simulink model "PONG"  (R2018b)
settings: Solver=VariableStepAuto  StartTime=0.0  StopTime=10  RelTol=1e-3
libraries: simulink_extras x28
(part 1 of 3)
settings Model: SimulationMode=accelerator  NumberOfSteps=2  SnapshotBufferSize=100  SnapshotInterval=100  Creator=Baraghini Nicholas  LastModifiedBy=Baraghini Nicholas

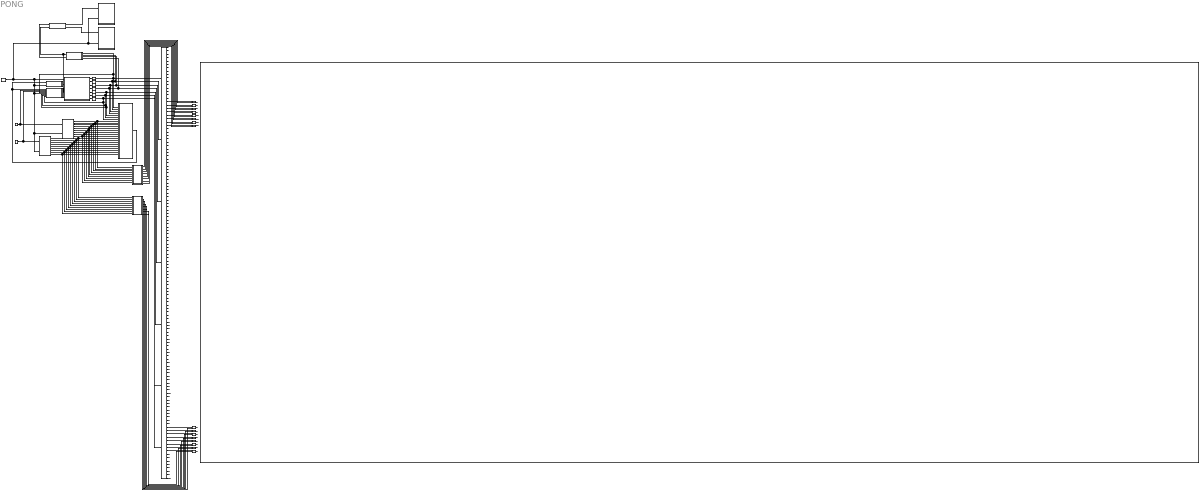
== system PONG ==
  Clock : simulink_extras/Flip Flops/Clock  period=1
  DECODER_7 bit : Subsystem  TreatAsAtomicUnit=on
  Horizontal Bounce : Subsystem  TreatAsAtomicUnit=on
  "LAMP_DISPLAY " : Subsystem  TreatAsAtomicUnit=on
  Logical Operator{,1..15} (16 alike) : Logic  Operator=OR  IconShape=distinctive  AllPortsSameDT=off  OutDataTypeStr=boolean
  Memory{,1..6} (7 alike) : Memory  InheritSampleTime=on
  "Next State " : Subsystem  TreatAsAtomicUnit=on
  Paddle Control : Subsystem  TreatAsAtomicUnit=on
  Paddle DEMUXER0 : Subsystem  TreatAsAtomicUnit=on
  Paddle DEMUXER1 : Subsystem  TreatAsAtomicUnit=on
  Paddle0 : Subsystem  TreatAsAtomicUnit=on
  Paddle1 : Subsystem  TreatAsAtomicUnit=on
  PointReset : Subsystem  TreatAsAtomicUnit=on
  Subsystem : Subsystem
  Subsystem2 : Subsystem
  Switch0 : Constant  OutDataTypeStr=boolean
  Switch1 : Constant  Value=0  OutDataTypeStr=boolean
  Vertical Bounce2 : Subsystem  TreatAsAtomicUnit=on
  Vertical Bounce3 : Subsystem  TreatAsAtomicUnit=on
  wires:
  "Next State "/1(A1) -> Memory6/1
  "Next State "/2(B1) -> Memory5/1
  "Next State "/3(C1) -> Memory4/1
  "Next State "/4(D1) -> Memory3/1
  "Next State "/5(E1) -> Memory2/1
  DECODER_7 bit/1(0000000) -> ?
  DECODER_7 bit/2("0000001 ") -> ?
  DECODER_7 bit/3(0000010) -> ?
  DECODER_7 bit/4(0000011) -> ?
  DECODER_7 bit/5(0000100) -> ?
  DECODER_7 bit/6(0000101) -> ?
  DECODER_7 bit/7(0000110) -> ?
  DECODER_7 bit/8(0000111) -> ?
  DECODER_7 bit/9(0001000) -> ?
  DECODER_7 bit/10(0001001) -> ?
  DECODER_7 bit/11(0001010) -> ?
  DECODER_7 bit/12(0001011) -> ?
  DECODER_7 bit/13(0001100) -> ?
  DECODER_7 bit/14(0001101) -> ?
  DECODER_7 bit/15(0001110) -> ?
  DECODER_7 bit/16(0001111) -> ?
  DECODER_7 bit/17(0010000) -> Logical Operator/1
  DECODER_7 bit/18(0010001) -> Logical Operator1/1
  DECODER_7 bit/19(0010010) -> Logical Operator2/1
  DECODER_7 bit/20(0010011) -> Logical Operator3/1
  DECODER_7 bit/21(0010100) -> Logical Operator4/1
  DECODER_7 bit/22(0010101) -> Logical Operator5/1
  DECODER_7 bit/23(0010110) -> Logical Operator6/1
  DECODER_7 bit/24(0010111) -> Logical Operator7/1
  DECODER_7 bit/25(0011000) -> ?
  DECODER_7 bit/26(0011001) -> ?
  DECODER_7 bit/27(0011010) -> ?
  DECODER_7 bit/28(0011011) -> ?
  DECODER_7 bit/29(0011100) -> ?
  DECODER_7 bit/30(0011101) -> ?
  DECODER_7 bit/31(0011110) -> ?
  DECODER_7 bit/32(0011111) -> ?
  DECODER_7 bit/33(0100000) -> ?
  DECODER_7 bit/34(0100001) -> ?
  DECODER_7 bit/35(0100010) -> ?
  DECODER_7 bit/36(0100011) -> ?
  DECODER_7 bit/37(0100100) -> ?
  DECODER_7 bit/38(0100110) -> ?
  DECODER_7 bit/39(0100111) -> ?
  DECODER_7 bit/40(0101000) -> ?
  DECODER_7 bit/41(0101001) -> ?
  DECODER_7 bit/42(0101010) -> ?
  DECODER_7 bit/43(0101011) -> ?
  DECODER_7 bit/44(0101100) -> ?
  DECODER_7 bit/45(0101101) -> ?
  DECODER_7 bit/46(0101110) -> ?
  DECODER_7 bit/47(0101111) -> ?
  DECODER_7 bit/48(0110000) -> ?
  DECODER_7 bit/49(0110001) -> ?
  DECODER_7 bit/50(0110010) -> ?
  DECODER_7 bit/51(0110011) -> ?
  DECODER_7 bit/52(0110100) -> ?
  DECODER_7 bit/53(0110101) -> ?
  DECODER_7 bit/54(0110110) -> ?
  DECODER_7 bit/55(0110111) -> ?
  DECODER_7 bit/56(0111000) -> ?
  DECODER_7 bit/57(0111001) -> ?
  DECODER_7 bit/58(0111010) -> ?
  DECODER_7 bit/59(0111011) -> ?
  DECODER_7 bit/60(0111100) -> ?
  DECODER_7 bit/61(0111101) -> ?
  DECODER_7 bit/62(0111110) -> ?
  DECODER_7 bit/63(0111111) -> ?
  DECODER_7 bit/64(0100101) -> ?
  DECODER_7 bit/65(1000000) -> ?
  DECODER_7 bit/66(1000001) -> ?
  DECODER_7 bit/67(1000010) -> ?
  DECODER_7 bit/68(1000011) -> ?
  DECODER_7 bit/69(1000100) -> ?
  DECODER_7 bit/70(1000101) -> ?
  DECODER_7 bit/71(1000110) -> ?
  DECODER_7 bit/72(1000111) -> ?
  DECODER_7 bit/73(1001000) -> ?
  DECODER_7 bit/74(1001001) -> ?
  DECODER_7 bit/75(1001010) -> ?
  DECODER_7 bit/76(1001011) -> ?
  DECODER_7 bit/77(1001100) -> ?
  DECODER_7 bit/78(1001101) -> ?
  DECODER_7 bit/79(1001110) -> ?
  DECODER_7 bit/80(1001111) -> ?
  DECODER_7 bit/81(1010000) -> ?
  DECODER_7 bit/82(1010001) -> ?
  DECODER_7 bit/83(1010010) -> ?
  DECODER_7 bit/84(1010011) -> ?
  DECODER_7 bit/85(1010100) -> ?
  DECODER_7 bit/86(1010101) -> ?
  DECODER_7 bit/87(1010110) -> ?
  DECODER_7 bit/88(1010111) -> ?
  DECODER_7 bit/89(1011000) -> ?
  DECODER_7 bit/90(1011001) -> ?
  DECODER_7 bit/91(1011010) -> ?
  DECODER_7 bit/92(1011011) -> ?
  DECODER_7 bit/113(1110000) -> Logical Operator8/1
  DECODER_7 bit/114(1110001) -> Logical Operator9/1
  DECODER_7 bit/115(1110010) -> Logical Operator10/1
  DECODER_7 bit/116(1110011) -> Logical Operator11/1
  DECODER_7 bit/117(1110100) -> Logical Operator12/1
  DECODER_7 bit/118(1110101) -> Logical Operator13/1
  DECODER_7 bit/119(1110110) -> Logical Operator14/1
  DECODER_7 bit/120(1110111) -> Logical Operator15/1
  Paddle0/1(PA) -> Paddle DEMUXER0/1(PA0), Paddle Control/8(PA)
  Paddle0/9(PC2) -> Paddle DEMUXER0/9(PC2), Paddle Control/16(PC2)
  Paddle0/8(PB2) -> Paddle DEMUXER0/8(PB2), Paddle Control/15(PB2)
  Paddle0/7(PA2) -> Paddle DEMUXER0/7(PA2), Paddle Control/14(PA2)
  Paddle0/2(PB) -> Paddle DEMUXER0/2(PB0), Paddle Control/9(PB)
  Paddle0/5(PB1) -> Paddle DEMUXER0/5(PB1), Paddle Control/12(PB1)
  Paddle1/1(PA) -> Paddle DEMUXER1/1(PA0), Paddle Control/17(1PA)
  Paddle1/3(PC) -> Paddle DEMUXER1/3(PC0), Paddle Control/19(1PC)
  Paddle1/4(PA1) -> Paddle DEMUXER1/4(PA1), Paddle Control/20(1PA1)
  Paddle1/5(PB1) -> Paddle DEMUXER1/5(PB1), Paddle Control/21(1PB1)
  Paddle1/9(PC2) -> Paddle DEMUXER1/9(PC2), Paddle Control/25(1PC2)
  Paddle Control/1(Check) -> Vertical Bounce3/1(Check), Horizontal Bounce/1(Check)
  "Next State "/6(F1) -> Memory1/1
  "Next State "/7(G1) -> Memory/1
  Paddle0/3(PC) -> Paddle DEMUXER0/3(PC0), Paddle Control/10(PC)
  Paddle0/4(PA1) -> Paddle DEMUXER0/4(PA1), Paddle Control/11(PA1)
  Paddle0/6(PC1) -> Paddle DEMUXER0/6(PC1), Paddle Control/13(PC1)
  Paddle1/2(PB) -> Paddle DEMUXER1/2(PB0), Paddle Control/18(1PB)
  Paddle1/6(PC1) -> Paddle DEMUXER1/6(PC1), Paddle Control/22(1PC1)
  Paddle1/7(PA2) -> Paddle DEMUXER1/7(PA2), Paddle Control/23(1PA2)
  Paddle1/8(PB2) -> Paddle DEMUXER1/8(PB2), Paddle Control/24(1PB2)
  Horizontal Bounce/1(HEnable) -> "Next State "/2(EN_Xball1)
  Switch0/1 -> Vertical Bounce3/2(Ctrl0), Paddle0/1(Controller)
  Switch1/1 -> Paddle1/1(Controller), Vertical Bounce3/3(Ctrl1)
  Logical Operator/1 -> ?
  Logical Operator8/1 -> ?
  Logical Operator9/1 -> ?
  Logical Operator10/1 -> ?
  Logical Operator11/1 -> ?
  Logical Operator12/1 -> ?
  Logical Operator13/1 -> ?
  Logical Operator14/1 -> ?
  Logical Operator15/1 -> ?
  Paddle DEMUXER0/1(000) -> Logical Operator/2
  Paddle DEMUXER0/2(001) -> Logical Operator1/2
  Paddle DEMUXER0/3(010) -> Logical Operator2/2
  Paddle DEMUXER0/4(011) -> Logical Operator3/2
  Paddle DEMUXER0/5(100) -> Logical Operator4/2
  Paddle DEMUXER0/6(101) -> Logical Operator5/2
  Paddle DEMUXER0/7(110) -> Logical Operator6/2
  Paddle DEMUXER0/8(111) -> Logical Operator7/2
  Paddle DEMUXER1/8(111) -> Logical Operator15/2
  Paddle DEMUXER1/7(110) -> Logical Operator14/2
  Paddle DEMUXER1/6(101) -> Logical Operator13/2
  Paddle DEMUXER1/1(000) -> Logical Operator8/2
  Paddle DEMUXER1/2(001) -> Logical Operator9/2
  Paddle DEMUXER1/3(010) -> Logical Operator10/2
  Paddle DEMUXER1/4(011) -> Logical Operator11/2
  Paddle DEMUXER1/5(100) -> Logical Operator12/2
  DECODER_7 bit/93("1011100 ") -> ?
  DECODER_7 bit/94(1011101) -> ?
  DECODER_7 bit/95(1011110) -> ?
  DECODER_7 bit/96(1011111) -> ?
  DECODER_7 bit/97(1100000) -> ?
  DECODER_7 bit/98(1100001) -> ?
  DECODER_7 bit/99(1100010) -> ?
  DECODER_7 bit/100(1100011) -> ?
  DECODER_7 bit/101(1100100) -> ?
  DECODER_7 bit/102(1100101) -> ?
  DECODER_7 bit/103(1100110) -> ?
  DECODER_7 bit/104(1100111) -> ?
  DECODER_7 bit/105(1101000) -> ?
  DECODER_7 bit/106(1101001) -> ?
  DECODER_7 bit/107(1101010) -> ?
  DECODER_7 bit/108(1101011) -> ?
  DECODER_7 bit/109(1101100) -> ?
  DECODER_7 bit/110(1101101) -> ?
  DECODER_7 bit/111(1101110) -> ?
  DECODER_7 bit/112(1101111) -> ?
  DECODER_7 bit/121(1111000) -> ?
  DECODER_7 bit/122(1111001) -> ?
  DECODER_7 bit/123(1111010) -> ?
  DECODER_7 bit/124(1111011) -> ?
  DECODER_7 bit/125(1111100) -> ?
  DECODER_7 bit/126(1111101) -> ?
  DECODER_7 bit/127(1111110) -> ?
  DECODER_7 bit/128(1111111) -> ?
  Logical Operator1/1 -> ?
  Logical Operator2/1 -> ?
  Logical Operator3/1 -> ?
  Logical Operator4/1 -> ?
  Logical Operator5/1 -> ?
  Logical Operator6/1 -> ?
  Logical Operator7/1 -> ?
  Vertical Bounce3/1(VEnable 1) -> "Next State "/3(EN_Yball1)
  Vertical Bounce3/2(VEnable 0) -> "Next State "/4(EN_Yball0)
  Memory/1 -> DECODER_7 bit/7(In7), Vertical Bounce3/8(G), Paddle Control/7(G)
  Memory1/1 -> DECODER_7 bit/6(In6), Vertical Bounce3/7(F), Paddle Control/6(F)
  Memory2/1 -> DECODER_7 bit/5(In5), Vertical Bounce3/6(E), Paddle Control/5(E)
  Memory3/1 -> PointReset/4(D), DECODER_7 bit/4(In4), Paddle Control/4(D)
  Memory4/1 -> PointReset/3(C), DECODER_7 bit/3(In3), Paddle Control/3(C)
  Memory5/1 -> DECODER_7 bit/2(In2), PointReset/2(B), Paddle Control/2(B)
  Memory6/1 -> Vertical Bounce3/4(A), PointReset/1(A), Paddle Control/1(A), DECODER_7 bit/1(In1)
  PointReset/1(PointReset) -> Vertical Bounce2/2(PointReset), "Next State "/5("EN_reset ")
  Vertical Bounce2/2(Point1) -> Subsystem2/1(EN)
  Vertical Bounce2/1(Point0) -> Subsystem/1(En)
  PointReset/2(Winner) -> Vertical Bounce2/1(Winner)
  Clock/1 -> Subsystem/2(CLK), Subsystem2/2(CLK), "Next State "/1(CLK 1), Paddle1/2(CLK), Paddle0/2(CLK), Vertical Bounce3/5(CLK), Horizontal Bounce/2(CLK)

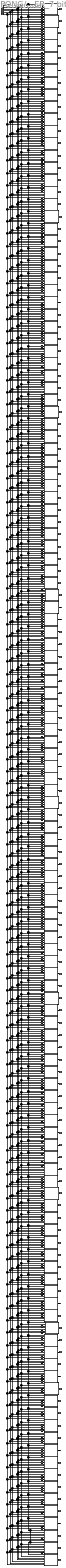
== system PONG/DECODER_7 bit ==
  In1 : Inport
  In2 : Inport  Port=2
  In3 : Inport  Port=3
  In4 : Inport  Port=4
  In5 : Inport  Port=5
  In6 : Inport  Port=6
  In7 : Inport  Port=7
  Logical Operator{,1..127} (128 alike) : Logic  Inputs=7  IconShape=distinctive  AllPortsSameDT=off  OutDataTypeStr=boolean
  NOT{,1..86,88..173,175..178,180..185,187..188,190..221,223..238,240..248,250..281,283..288,290,292..295,297..299,301,303..306,308..311,313..314,316,319..322,324..328,331..332,334..335,337..338,341..342,344,346,348..349,351,353..354,356..359,361..365,367..369,371..376,378..380,382..386,388,390..393,395,397..399,401..405,407..408,410,412..414,416..417,419..421,423..429,431,433..434,436..442,444..447,449..453,455..456,458..463,465..468,470..474,476..478,480..481,483..484,486..488,490..493,495,497..504,506..509,511..513} (448 alike) : Logic  Operator=NOT  IconShape=distinctive  AllPortsSameDT=off  OutDataTypeStr=boolean
  0000000 : Outport
  "0000001 " : Outport  Port=2
  0000010 : Outport  Port=3
  0000011 : Outport  Port=4
  0000100 : Outport  Port=5
  0000101 : Outport  Port=6
  0000110 : Outport  Port=7
  0000111 : Outport  Port=8
  0001000 : Outport  Port=9
  0001001 : Outport  Port=10
  0001010 : Outport  Port=11
  0001011 : Outport  Port=12
  0001100 : Outport  Port=13
  0001101 : Outport  Port=14
  0001110 : Outport  Port=15
  0001111 : Outport  Port=16
  0010000 : Outport  Port=17
  0010001 : Outport  Port=18
  0010010 : Outport  Port=19
  0010011 : Outport  Port=20
  0010100 : Outport  Port=21
  0010101 : Outport  Port=22
  0010110 : Outport  Port=23
  0010111 : Outport  Port=24
  0011000 : Outport  Port=25
  0011001 : Outport  Port=26
  0011010 : Outport  Port=27
  0011011 : Outport  Port=28
  0011100 : Outport  Port=29
  0011101 : Outport  Port=30
  0011110 : Outport  Port=31
  0011111 : Outport  Port=32
  0100000 : Outport  Port=33
  0100001 : Outport  Port=34
  0100010 : Outport  Port=35
  0100011 : Outport  Port=36
  0100100 : Outport  Port=37
  0100110 : Outport  Port=38
  0100111 : Outport  Port=39
  0101000 : Outport  Port=40
  0101001 : Outport  Port=41
  0101010 : Outport  Port=42
  0101011 : Outport  Port=43
  0101100 : Outport  Port=44
  0101101 : Outport  Port=45
  0101110 : Outport  Port=46
  0101111 : Outport  Port=47
  0110000 : Outport  Port=48
  0110001 : Outport  Port=49
  0110010 : Outport  Port=50
  0110011 : Outport  Port=51
  0110100 : Outport  Port=52
  0110101 : Outport  Port=53
  0110110 : Outport  Port=54
  0110111 : Outport  Port=55
  0111000 : Outport  Port=56
  0111001 : Outport  Port=57
  0111010 : Outport  Port=58
  0111011 : Outport  Port=59
  0111100 : Outport  Port=60
  0111101 : Outport  Port=61
  0111110 : Outport  Port=62
  0111111 : Outport  Port=63
  0100101 : Outport  Port=64
  1000000 : Outport  Port=65
  1000001 : Outport  Port=66
  1000010 : Outport  Port=67
  1000011 : Outport  Port=68
  1000100 : Outport  Port=69
  1000101 : Outport  Port=70
  1000110 : Outport  Port=71
  1000111 : Outport  Port=72
  1001000 : Outport  Port=73
  1001001 : Outport  Port=74
  1001010 : Outport  Port=75
  1001011 : Outport  Port=76
  1001100 : Outport  Port=77
  1001101 : Outport  Port=78
  1001110 : Outport  Port=79
  1001111 : Outport  Port=80
  1010000 : Outport  Port=81
  1010001 : Outport  Port=82
  1010010 : Outport  Port=83
  1010011 : Outport  Port=84
  1010100 : Outport  Port=85
  1010101 : Outport  Port=86
  1010110 : Outport  Port=87
  1010111 : Outport  Port=88
  1011000 : Outport  Port=89
  1011001 : Outport  Port=90
  1011010 : Outport  Port=91
  1011011 : Outport  Port=92
  "1011100 " : Outport  Port=93
  1011101 : Outport  Port=94
  1011110 : Outport  Port=95
  1011111 : Outport  Port=96
  1100000 : Outport  Port=97
  1100001 : Outport  Port=98
  1100010 : Outport  Port=99
  1100011 : Outport  Port=100
  1100100 : Outport  Port=101
  1100101 : Outport  Port=102
  1100110 : Outport  Port=103
  1100111 : Outport  Port=104
  1101000 : Outport  Port=105
  1101001 : Outport  Port=106
  1101010 : Outport  Port=107
  1101011 : Outport  Port=108
  1101100 : Outport  Port=109
  1101101 : Outport  Port=110
  1101110 : Outport  Port=111
  1101111 : Outport  Port=112
  1110000 : Outport  Port=113
  1110001 : Outport  Port=114
  1110010 : Outport  Port=115
  1110011 : Outport  Port=116
  1110100 : Outport  Port=117
  1110101 : Outport  Port=118
  1110110 : Outport  Port=119
  1110111 : Outport  Port=120
  1111000 : Outport  Port=121
  1111001 : Outport  Port=122
  1111010 : Outport  Port=123
  1111011 : Outport  Port=124
  1111100 : Outport  Port=125
  1111101 : Outport  Port=126
  1111110 : Outport  Port=127
  1111111 : Outport  Port=128
  wires:
  NOT/1 -> Logical Operator/1
  NOT1/1 -> Logical Operator/2
  NOT2/1 -> Logical Operator/3
  NOT3/1 -> Logical Operator/4
  NOT4/1 -> Logical Operator/5
  NOT5/1 -> Logical Operator/6
  NOT6/1 -> Logical Operator/7
  NOT7/1 -> Logical Operator1/1
  NOT8/1 -> Logical Operator1/2
  NOT9/1 -> Logical Operator1/3
  NOT10/1 -> Logical Operator1/4
  NOT11/1 -> Logical Operator1/5
  NOT12/1 -> Logical Operator1/6
  NOT17/1 -> Logical Operator2/5
  NOT13/1 -> Logical Operator2/1
  NOT14/1 -> Logical Operator2/2
  NOT15/1 -> Logical Operator2/3
  NOT16/1 -> Logical Operator2/4
  NOT19/1 -> Logical Operator2/7
  NOT23/1 -> Logical Operator3/5
  NOT18/1 -> Logical Operator3/1
  NOT20/1 -> Logical Operator3/2
  NOT21/1 -> Logical Operator3/3
  NOT22/1 -> Logical Operator3/4
  In7/1 -> Logical Operator1/7, NOT19/1, Logical Operator7/7, NOT50/1, NOT61/1, Logical Operator11/7, Logical Operator13/7, Logical Operator15/7, Logical Operator26/7, Logical Operator28/7, Logical Operator30/7, NOT132/1, NOT144/1, Logical Operator20/7, NOT163/1, Logical Operator54/7, Logical Operator59/7, Logical Operator35/7, Logical Operator37/7, Logical Operator39/7, NOT286/1, Logical Operator52/7, NOT165/1, NOT173/1, NOT183/1, Logical Operator44/7, NOT192/1, Logical Operator48/7, Logical Operator65/7, Logical Operator87/7, NOT451/1, Logical Operator67/7, NOT492/1, NOT500/1, Logical Operator74/7, Logical Operator83/7, NOT267/1, Logical Operator90/7, Logical Operator77/7, NOT316/1, Logical Operator79/7, NOT325/1, Logical Operator81/7, NOT402/1, NOT327/1, Logical Operator115/7, Logical Operator117/7, Logical Operator105/7, NOT356/1, Logical Operator107/7, NOT351/1, Logical Operator103/7, NOT342/1, NOT335/1, Logical Operator112/7, NOT288/1, Logical Operator110/7, NOT436/1, Logical Operator100/7, NOT426/1, Logical Operator97/7, NOT420/1, Logical Operator95/7, NOT413/1, Logical Operator93/7, NOT404/1, Logical Operator124/7, NOT393/1, Logical Operator122/7, NOT383/1, Logical Operator119/7, NOT373/1, Logical Operator114/7, NOT361/1, Logical Operator91/7, NOT306/1, NOT293/1, Logical Operator88/7, Logical Operator85/7, NOT200/1, NOT511/1, Logical Operator71/7, Logical Operator69/7, NOT483/1, NOT473/1, Logical Operator127/7, NOT461/1, Logical Operator125/7, Logical Operator109/7, NOT439/1, NOT348/1, NOT471/1, NOT199/1, Logical Operator46/7, Logical Operator57/7, Logical Operator55/7, NOT127/1, Logical Operator50/7, Logical Operator41/7, NOT276/1, NOT269/1, NOT260/1, NOT250/1, Logical Operator63/7, NOT238/1, Logical Operator61/7, NOT228/1, NOT216/1, NOT203/1, Logical Operator33/7, NOT248/1, Logical Operator24/7, Logical Operator22/7, NOT154/1, Logical Operator32/7, NOT122/1, NOT110/1, NOT97/1, Logical Operator18/7, NOT86/1, NOT79/1, NOT70/1, Logical Operator9/7, NOT41/1, Logical Operator5/7, NOT30/1, Logical Operator3/7, NOT6/1
  NOT25/1 -> Logical Operator4/2
  NOT26/1 -> Logical Operator4/3
  NOT27/1 -> Logical Operator4/4
  NOT24/1 -> Logical Operator4/1
  NOT29/1 -> Logical Operator4/6
  NOT30/1 -> Logical Operator4/7
  NOT31/1 -> Logical Operator5/2
  NOT32/1 -> Logical Operator5/3
  NOT33/1 -> Logical Operator5/4
  NOT28/1 -> Logical Operator5/1
  NOT35/1 -> Logical Operator5/6
  NOT36/1 -> Logical Operator6/2
  NOT37/1 -> Logical Operator6/3
  NOT38/1 -> Logical Operator6/4
  NOT34/1 -> Logical Operator6/1
  NOT41/1 -> Logical Operator6/7
  NOT40/1 -> Logical Operator7/2
  NOT42/1 -> Logical Operator7/3
  NOT43/1 -> Logical Operator7/4
  NOT39/1 -> Logical Operator7/1
  NOT45/1 -> Logical Operator8/2
  NOT46/1 -> Logical Operator8/3
  NOT48/1 -> Logical Operator8/5
  NOT44/1 -> Logical Operator8/1
  NOT49/1 -> Logical Operator8/6
  NOT50/1 -> Logical Operator8/7
  NOT51/1 -> Logical Operator9/2
  NOT52/1 -> Logical Operator9/3
  NOT54/1 -> Logical Operator9/5
  NOT47/1 -> Logical Operator9/1
  NOT55/1 -> Logical Operator9/6
  NOT56/1 -> Logical Operator10/2
  NOT57/1 -> Logical Operator10/3
  NOT59/1 -> Logical Operator10/5
  NOT53/1 -> Logical Operator10/1
  NOT61/1 -> Logical Operator10/7
  NOT60/1 -> Logical Operator11/2
  NOT62/1 -> Logical Operator11/3
  NOT64/1 -> Logical Operator11/5
  NOT58/1 -> Logical Operator11/1
  NOT65/1 -> Logical Operator12/2
  NOT66/1 -> Logical Operator12/3
  NOT63/1 -> Logical Operator12/1
  NOT69/1 -> Logical Operator12/6
  NOT70/1 -> Logical Operator12/7
  NOT68/1 -> Logical Operator13/2
  NOT71/1 -> Logical Operator13/3
  NOT67/1 -> Logical Operator13/1
  NOT74/1 -> Logical Operator13/6
  NOT73/1 -> Logical Operator14/2
  NOT75/1 -> Logical Operator14/3
  NOT72/1 -> Logical Operator14/1
  NOT79/1 -> Logical Operator14/7
  NOT77/1 -> Logical Operator15/2
  NOT78/1 -> Logical Operator15/3
  NOT76/1 -> Logical Operator15/1
  NOT81/1 -> Logical Operator16/2
  NOT83/1 -> Logical Operator16/4
  NOT84/1 -> Logical Operator16/5
  NOT80/1 -> Logical Operator16/1
  NOT85/1 -> Logical Operator16/6
  NOT86/1 -> Logical Operator16/7
  NOT97/1 -> Logical Operator25/7
  NOT89/1 -> Logical Operator18/5
  NOT160/1 -> Logical Operator24/1
  NOT144/1 -> Logical Operator19/7
  NOT135/1 -> Logical Operator19/1
  NOT141/1 -> Logical Operator19/5
  NOT138/1 -> Logical Operator19/2
  NOT150/1 -> Logical Operator22/1
  NOT161/1 -> Logical Operator24/2
  NOT151/1 -> Logical Operator22/2
  NOT163/1 -> Logical Operator23/7
  NOT156/1 -> Logical Operator23/1
  NOT158/1 -> Logical Operator22/6
  NOT137/1 -> Logical Operator32/6
  NOT128/1 -> Logical Operator32/1
  NOT136/1 -> Logical Operator32/5
  NOT133/1 -> Logical Operator32/2
  NOT132/1 -> Logical Operator31/7
  NOT125/1 -> Logical Operator31/1
  NOT129/1 -> Logical Operator31/5
  NOT115/1 -> Logical Operator28/6
  NOT107/1 -> Logical Operator28/1
  NOT147/1 -> Logical Operator20/5
  NOT143/1 -> Logical Operator20/2
  NOT146/1 -> Logical Operator21/1
  NOT122/1 -> Logical Operator29/7
  NOT88/1 -> Logical Operator18/4
  NOT113/1 -> Logical Operator28/4
  NOT126/1 -> Logical Operator31/2
  NOT104/1 -> Logical Operator27/2
  NOT110/1 -> Logical Operator27/7
  NOT108/1 -> Logical Operator27/6
  NOT140/1 -> Logical Operator20/1
  NOT103/1 -> Logical Operator27/1
  NOT99/1 -> Logical Operator26/2
  NOT111/1 -> Logical Operator28/2
  NOT101/1 -> Logical Operator26/4
  NOT96/1 -> Logical Operator26/1
  NOT114/1 -> Logical Operator29/1
  NOT157/1 -> Logical Operator23/2
  NOT118/1 -> Logical Operator29/4
  NOT102/1 -> Logical Operator26/5
  NOT116/1 -> Logical Operator29/2
  NOT90/1 -> Logical Operator18/6
  NOT164/1 -> Logical Operator18/2
  NOT94/1 -> Logical Operator25/4
  NOT91/1 -> Logical Operator25/1
  NOT92/1 -> Logical Operator25/2
  NOT95/1 -> Logical Operator25/5
  NOT152/1 -> Logical Operator21/6
  NOT148/1 -> Logical Operator21/2
  NOT130/1 -> Logical Operator31/6
  NOT121/1 -> Logical Operator30/2
  NOT154/1 -> Logical Operator21/7
  NOT124/1 -> Logical Operator30/4
  NOT153/1 -> Logical Operator18/1
  NOT119/1 -> Logical Operator30/1
  NOT106/1 -> Logical Operator27/4
  NOT203/1 -> Logical Operator43/7
  NOT226/1 -> Logical Operator17/5
  NOT276/1 -> Logical Operator40/7
  NOT273/1 -> Logical Operator40/4
  NOT266/1 -> Logical Operator39/1
  NOT274/1 -> Logical Operator40/5
  NOT117/1 -> Logical Operator52/1
  NOT185/1 -> Logical Operator44/5
  NOT142/1 -> Logical Operator52/6
  NOT176/1 -> Logical Operator57/5
  NOT177/1 -> Logical Operator57/6
  NOT169/1 -> Logical Operator57/1
  NOT188/1 -> Logical Operator46/1
  NOT175/1 -> Logical Operator42/1
  NOT183/1 -> Logical Operator42/7
  NOT181/1 -> Logical Operator42/5
  NOT237/1 -> Logical Operator17/6
  NOT197/1 -> Logical Operator48/1
  NOT278/1 -> Logical Operator41/5
  NOT286/1 -> Logical Operator49/7
  NOT155/1 -> Logical Operator55/1
  NOT166/1 -> Logical Operator55/4
  NOT123/1 -> Logical Operator33/5
  NOT192/1 -> Logical Operator45/7
  NOT190/1 -> Logical Operator45/6
  NOT284/1 -> Logical Operator49/5
  NOT281/1 -> Logical Operator49/1
  NOT280/1 -> Logical Operator41/6
  NOT100/1 -> Logical Operator50/5
  NOT283/1 -> Logical Operator49/4
  NOT172/1 -> Logical Operator56/6
  NOT139/1 -> Logical Operator53/1
  NOT285/1 -> Logical Operator50/1
  NOT184/1 -> Logical Operator45/1
  NOT105/1 -> Logical Operator51/1
  NOT165/1 -> Logical Operator53/7
  NOT127/1 -> Logical Operator51/7
  NOT277/1 -> Logical Operator41/4
  NOT120/1 -> Logical Operator51/6
  NOT134/1 -> Logical Operator52/4
  NOT245/1 -> Logical Operator34/3
  NOT250/1 -> Logical Operator34/7
  NOT241/1 -> Logical Operator34/1
  NOT247/1 -> Logical Operator34/5
  NOT193/1 -> Logical Operator47/1
  NOT256/1 -> Logical Operator37/1
  NOT261/1 -> Logical Operator37/3
  NOT265/1 -> Logical Operator38/3
  NOT269/1 -> Logical Operator38/7
  NOT262/1 -> Logical Operator38/1
  NOT264/1 -> Logical Operator37/6
  NOT243/1 -> Logical Operator63/6
  NOT234/1 -> Logical Operator63/1
  NOT149/1 -> Logical Operator53/4
  NOT242/1 -> Logical Operator63/5
  NOT199/1 -> Logical Operator47/7
  NOT238/1 -> Logical Operator62/7
  NOT231/1 -> Logical Operator62/1
  NOT235/1 -> Logical Operator62/5
  NOT233/1 -> Logical Operator62/3
  NOT98/1 -> Logical Operator50/4
  NOT240/1 -> Logical Operator63/3
  NOT221/1 -> Logical Operator59/6
  NOT213/1 -> Logical Operator59/1
  NOT253/1 -> Logical Operator35/5
  NOT252/1 -> Logical Operator36/1
  NOT228/1 -> Logical Operator60/7
  NOT93/1 -> Logical Operator33/4
  NOT219/1 -> Logical Operator59/4
  NOT191/1 -> Logical Operator41/1
  NOT216/1 -> Logical Operator58/7
  NOT214/1 -> Logical Operator58/6
  NOT246/1 -> Logical Operator35/1
  NOT209/1 -> Logical Operator58/1
  NOT180/1 -> Logical Operator44/1
  NOT279/1 -> Logical Operator33/3
  NOT211/1 -> Logical Operator58/3
  NOT206/1 -> Logical Operator54/3
  NOT112/1 -> Logical Operator51/4
  NOT207/1 -> Logical Operator54/4
  NOT202/1 -> Logical Operator54/1
  NOT82/1 -> Logical Operator17/1
  NOT220/1 -> Logical Operator60/1
  NOT224/1 -> Logical Operator60/4
  NOT223/1 -> Logical Operator60/3
  NOT208/1 -> Logical Operator54/5
  NOT159/1 -> Logical Operator33/6
  NOT173/1 -> Logical Operator56/7
  NOT196/1 -> Logical Operator43/4
  NOT195/1 -> Logical Operator46/6
  NOT251/1 -> Logical Operator35/3
  NOT271/1 -> Logical Operator40/1
  NOT171/1 -> Logical Operator43/1
  NOT268/1 -> Logical Operator39/3
  NOT218/1 -> Logical Operator59/3
  NOT201/1 -> Logical Operator43/5
  NOT248/1 -> Logical Operator17/7
  NOT255/1 -> Logical Operator36/3
  NOT258/1 -> Logical Operator36/6
  NOT236/1 -> Logical Operator62/6
  NOT229/1 -> Logical Operator61/3
  NOT275/1 -> Logical Operator40/6
  NOT260/1 -> Logical Operator36/7
  NOT230/1 -> Logical Operator61/4
  NOT259/1 -> Logical Operator33/1
  NOT170/1 -> Logical Operator56/5
  NOT204/1 -> Logical Operator17/3
  NOT187/1 -> Logical Operator43/3
  NOT215/1 -> Logical Operator17/4
  NOT225/1 -> Logical Operator61/1
  NOT212/1 -> Logical Operator58/4
  NOT167/1 -> Logical Operator56/1
  NOT449/1 -> Logical Operator64/5
  NOT498/1 -> Logical Operator72/5
  NOT337/1 -> Logical Operator117/5
  In1/1 -> NOT/1, NOT7/1, Logical Operator70/1, Logical Operator71/1, Logical Operator72/1, Logical Operator74/1, Logical Operator82/1, Logical Operator83/1, Logical Operator84/1, Logical Operator85/1, Logical Operator86/1, Logical Operator88/1, Logical Operator89/1, Logical Operator77/1, Logical Operator78/1, Logical Operator79/1, Logical Operator80/1, Logical Operator81/1, Logical Operator73/1, Logical Operator91/1, Logical Operator102/1, Logical Operator114/1, Logical Operator118/1, Logical Operator119/1, Logical Operator122/1, Logical Operator123/1, Logical Operator124/1, Logical Operator92/1, Logical Operator93/1, Logical Operator94/1, Logical Operator95/1, Logical Operator96/1, Logical Operator97/1, Logical Operator99/1, Logical Operator100/1, Logical Operator108/1, Logical Operator110/1, Logical Operator111/1, Logical Operator112/1, Logical Operator113/1, Logical Operator117/1, Logical Operator101/1, Logical Operator103/1, Logical Operator104/1, Logical Operator107/1, Logical Operator106/1, Logical Operator105/1, Logical Operator116/1, Logical Operator115/1, Logical Operator121/1, Logical Operator75/1, Logical Operator90/1, Logical Operator69/1, Logical Operator68/1, Logical Operator67/1, Logical Operator66/1, Logical Operator127/1, Logical Operator126/1, Logical Operator125/1, Logical Operator120/1, Logical Operator109/1, Logical Operator98/1, Logical Operator87/1, Logical Operator76/1, Logical Operator65/1, Logical Operator64/1, NOT197/1, NOT193/1, NOT188/1, NOT184/1, NOT180/1, NOT175/1, NOT169/1, NOT167/1, NOT155/1, NOT139/1, NOT117/1, NOT105/1, NOT285/1, NOT281/1, NOT191/1, NOT271/1, NOT266/1, NOT262/1, NOT256/1, NOT252/1, NOT246/1, NOT241/1, NOT234/1, NOT231/1, NOT225/1, NOT220/1, NOT213/1, NOT209/1, NOT202/1, NOT171/1, NOT259/1, NOT82/1, NOT160/1, NOT156/1, NOT150/1, NOT146/1, NOT140/1, NOT135/1, NOT128/1, NOT125/1, NOT119/1, NOT114/1, NOT107/1, NOT103/1, NOT96/1, NOT91/1, NOT153/1, NOT80/1, NOT76/1, NOT72/1, NOT67/1, NOT63/1, NOT58/1, NOT53/1, NOT47/1, NOT44/1, NOT39/1, NOT34/1, NOT28/1, NOT24/1, NOT18/1, NOT13/1
  NOT497/1 -> Logical Operator72/4
  NOT401/1 -> Logical Operator92/5
  NOT404/1 -> Logical Operator92/7
  NOT427/1 -> Logical Operator100/4
  NOT288/1 -> Logical Operator111/7
  NOT327/1 -> Logical Operator113/7
  NOT433/1 -> Logical Operator108/4
  NOT145/1 -> Logical Operator110/5
  NOT431/1 -> Logical Operator100/6
  NOT434/1 -> Logical Operator108/5
  NOT351/1 -> Logical Operator104/7
  In2/1 -> NOT8/1, NOT14/1, NOT20/1, NOT25/1, NOT36/1, NOT40/1, NOT45/1, NOT51/1, NOT60/1, NOT65/1, NOT68/1, NOT73/1, NOT77/1, NOT81/1, NOT164/1, NOT92/1, NOT99/1, NOT116/1, NOT126/1, NOT133/1, NOT143/1, NOT148/1, NOT151/1, NOT157/1, NOT161/1, Logical Operator17/2, Logical Operator33/2, Logical Operator43/2, Logical Operator54/2, Logical Operator58/2, Logical Operator59/2, Logical Operator61/2, Logical Operator36/2, Logical Operator38/2, Logical Operator40/2, Logical Operator49/2, Logical Operator52/2, Logical Operator53/2, Logical Operator55/2, Logical Operator56/2, Logical Operator57/2, Logical Operator44/2, Logical Operator45/2, Logical Operator46/2, Logical Operator47/2, Logical Operator48/2, NOT109/1, NOT493/1, NOT301/1, NOT358/1, NOT403/1, NOT440/1, NOT445/1, NOT450/1, NOT455/1, NOT462/1, NOT467/1, NOT472/1, NOT477/1, NOT480/1, NOT486/1, NOT490/1, NOT495/1, NOT326/1, NOT506/1, NOT513/1, NOT178/1, NOT232/1, NOT263/1, NOT287/1, NOT305/1, NOT309/1, NOT313/1, NOT319/1, NOT324/1, Logical Operator73/2, Logical Operator91/2, Logical Operator102/2, Logical Operator114/2, Logical Operator122/2, Logical Operator123/2, Logical Operator92/2, Logical Operator93/2, Logical Operator94/2, Logical Operator95/2, Logical Operator96/2, Logical Operator97/2, Logical Operator99/2, Logical Operator100/2, Logical Operator108/2, Logical Operator110/2, Logical Operator111/2, Logical Operator112/2, Logical Operator113/2, Logical Operator115/2, Logical Operator116/2, Logical Operator117/2, Logical Operator101/2, Logical Operator103/2, Logical Operator104/2, Logical Operator105/2, Logical Operator107/2, Logical Operator106/2, Logical Operator124/2, Logical Operator121/2, Logical Operator119/2, Logical Operator118/2, NOT299/1, NOT294/1, NOT205/1, Logical Operator42/2, Logical Operator51/2, Logical Operator50/2, Logical Operator41/2, Logical Operator39/2, Logical Operator37/2, Logical Operator35/2, Logical Operator34/2, Logical Operator63/2, Logical Operator62/2, Logical Operator60/2, NOT138/1, NOT121/1, NOT111/1, NOT104/1, NOT56/1, NOT31/1, NOT1/1
  NOT341/1 -> Logical Operator101/5
  NOT334/1 -> Logical Operator116/6
  NOT392/1 -> Logical Operator73/6
  NOT305/1 -> Logical Operator77/2
  NOT297/1 -> Logical Operator90/5
  NOT298/1 -> Logical Operator90/6
  NOT324/1 -> Logical Operator81/2
  NOT306/1 -> Logical Operator75/7
  NOT299/1 -> Logical Operator75/2
  NOT303/1 -> Logical Operator75/5
  NOT460/1 -> Logical Operator64/6
  NOT272/1 -> Logical Operator88/4
  NOT198/1 -> Logical Operator65/5
  NOT316/1 -> Logical Operator78/7
  NOT263/1 -> Logical Operator88/2
  NOT495/1 -> Logical Operator72/2
  NOT309/1 -> Logical Operator78/2
  NOT314/1 -> Logical Operator78/6
  NOT509/1 -> Logical Operator82/5
  NOT504/1 -> Logical Operator74/6
  NOT168/1 -> Logical Operator83/5
  NOT508/1 -> Logical Operator82/4
  NOT292/1 -> Logical Operator89/6
  NOT319/1 -> Logical Operator80/2
  NOT232/1 -> Logical Operator86/2
  NOT295/1 -> Logical Operator112/4
  NOT513/1 -> Logical Operator83/2
  NOT205/1 -> Logical Operator85/2
  NOT270/1 -> Logical Operator91/5
  NOT267/1 -> Logical Operator86/7
  NOT200/1 -> Logical Operator84/7
  NOT501/1 -> Logical Operator74/4
  NOT217/1 -> Logical Operator85/4
  NOT287/1 -> Logical Operator89/2
  NOT468/1 -> Logical Operator66/3
  NOT473/1 -> Logical Operator66/7
  NOT470/1 -> Logical Operator66/5
  NOT467/1 -> Logical Operator66/2
  NOT484/1 -> Logical Operator69/3
  NOT490/1 -> Logical Operator71/2
  NOT480/1 -> Logical Operator69/2
  NOT436/1 -> Logical Operator108/7
  NOT492/1 -> Logical Operator70/7
  NOT487/1 -> Logical Operator69/6
  In5/1 -> NOT17/1, NOT23/1, Logical Operator4/5, Logical Operator6/5, Logical Operator7/5, NOT48/1, NOT54/1, NOT59/1, NOT64/1, Logical Operator12/5, Logical Operator15/5, NOT89/1, NOT102/1, Logical Operator27/5, Logical Operator29/5, Logical Operator21/5, Logical Operator24/5, NOT226/1, NOT201/1, NOT208/1, Logical Operator60/5, Logical Operator61/5, NOT235/1, NOT253/1, Logical Operator36/5, Logical Operator37/5, Logical Operator38/5, Logical Operator39/5, NOT274/1, NOT278/1, NOT100/1, Logical Operator51/5, Logical Operator52/5, Logical Operator53/5, NOT170/1, NOT176/1, NOT181/1, NOT185/1, Logical Operator45/5, Logical Operator46/5, Logical Operator47/5, NOT449/1, NOT198/1, NOT331/1, Logical Operator98/5, Logical Operator120/5, Logical Operator125/5, NOT458/1, NOT465/1, NOT470/1, NOT476/1, Logical Operator68/5, Logical Operator69/5, Logical Operator71/5, NOT509/1, NOT168/1, Logical Operator85/5, Logical Operator88/5, NOT297/1, NOT303/1, NOT308/1, Logical Operator78/5, Logical Operator81/5, NOT382/1, NOT270/1, NOT359/1, NOT365/1, Logical Operator119/5, Logical Operator121/5, Logical Operator122/5, NOT390/1, NOT397/1, NOT401/1, Logical Operator95/5, Logical Operator96/5, Logical Operator97/5, NOT424/1, NOT428/1, NOT434/1, Logical Operator111/5, Logical Operator113/5, Logical Operator115/5, NOT341/1, NOT344/1, Logical Operator104/5, Logical Operator105/5, Logical Operator107/5, Logical Operator106/5, NOT337/1, NOT332/1, Logical Operator112/5, NOT145/1, Logical Operator94/5, NOT407/1, Logical Operator118/5, Logical Operator80/5, Logical Operator79/5, NOT290/1, Logical Operator86/5, Logical Operator84/5, NOT502/1, NOT498/1, Logical Operator70/5, Logical Operator109/5, NOT385/1, Logical Operator48/5, Logical Operator55/5, NOT284/1, NOT247/1, NOT242/1, Logical Operator59/5, Logical Operator58/5, NOT123/1, Logical Operator23/5, Logical Operator22/5, NOT147/1, NOT141/1, NOT136/1, NOT129/1, Logical Operator30/5, Logical Operator28/5, NOT95/1, NOT84/1, Logical Operator14/5, Logical Operator13/5, Logical Operator5/5, NOT11/1, NOT4/1
  NOT294/1 -> Logical Operator90/2
  NOT413/1 -> Logical Operator94/7
  NOT428/1 -> Logical Operator100/5
  NOT425/1 -> Logical Operator99/6
  NOT391/1 -> Logical Operator123/6
  NOT408/1 -> Logical Operator94/3
  NOT402/1 -> Logical Operator73/7
  NOT359/1 -> Logical Operator102/5
  NOT374/1 -> Logical Operator119/3
  NOT328/1 -> Logical Operator115/4
  NOT419/1 -> Logical Operator97/3
  NOT349/1 -> Logical Operator104/6
  NOT354/1 -> Logical Operator102/4
  NOT353/1 -> Logical Operator105/6
  NOT502/1 -> Logical Operator74/5
  NOT321/1 -> Logical Operator91/6
  NOT335/1 -> Logical Operator116/7
  NOT379/1 -> Logical Operator121/3
  NOT380/1 -> Logical Operator121/4
  NOT365/1 -> Logical Operator114/5
  NOT210/1 -> Logical Operator111/4
  NOT363/1 -> Logical Operator114/3
  NOT371/1 -> Logical Operator118/6
  NOT507/1 -> Logical Operator91/4
  NOT375/1 -> Logical Operator119/4
  NOT383/1 -> Logical Operator121/7
  NOT342/1 -> Logical Operator101/7
  NOT348/1 -> Logical Operator76/7
  NOT395/1 -> Logical Operator124/3
  NOT378/1 -> Logical Operator119/6
  NOT407/1 -> Logical Operator93/5
  NOT512/1 -> Logical Operator110/4
  NOT326/1 -> Logical Operator74/2
  NOT390/1 -> Logical Operator123/5
  NOT393/1 -> Logical Operator123/7
  NOT308/1 -> Logical Operator77/5
  NOT398/1 -> Logical Operator124/6
  NOT356/1 -> Logical Operator106/7
  NOT488/1 -> Logical Operator70/3
  NOT397/1 -> Logical Operator124/5
  NOT310/1 -> Logical Operator113/4
  NOT420/1 -> Logical Operator96/7
  NOT417/1 -> Logical Operator96/3
  NOT429/1 -> Logical Operator91/3
  NOT257/1 -> Logical Operator111/6
  NOT368/1 -> Logical Operator118/3
  NOT466/1 -> Logical Operator127/6
  NOT244/1 -> Logical Operator86/4
  NOT465/1 -> Logical Operator127/5
  NOT325/1 -> Logical Operator80/7
  NOT462/1 -> Logical Operator127/2
  NOT461/1 -> Logical Operator126/7
  NOT458/1 -> Logical Operator126/5
  NOT455/1 -> Logical Operator126/2
  NOT386/1 -> Logical Operator122/4
  NOT456/1 -> Logical Operator126/3
  NOT162/1 -> Logical Operator83/4
  NOT442/1 -> Logical Operator109/4
  NOT463/1 -> Logical Operator127/3
  NOT444/1 -> Logical Operator109/6
  NOT440/1 -> Logical Operator109/2
  NOT182/1 -> Logical Operator84/4
  NOT474/1 -> Logical Operator67/3
  NOT476/1 -> Logical Operator67/5
  NOT338/1 -> Logical Operator117/6
  NOT472/1 -> Logical Operator67/2
  NOT399/1 -> Logical Operator92/3
  NOT414/1 -> Logical Operator95/3
  NOT451/1 -> Logical Operator120/7
  NOT503/1 -> Logical Operator65/3
  NOT131/1 -> Logical Operator65/4
  NOT477/1 -> Logical Operator68/2
  NOT459/1 -> Logical Operator126/6
  NOT478/1 -> Logical Operator68/3
  NOT439/1 -> Logical Operator98/7
  NOT437/1 -> Logical Operator98/6
  NOT388/1 -> Logical Operator123/3
  NOT358/1 -> Logical Operator87/2
  NOT412/1 -> Logical Operator98/3
  NOT367/1 -> Logical Operator87/3
  NOT382/1 -> Logical Operator73/5
  NOT361/1 -> Logical Operator102/7
  NOT194/1 -> Logical Operator84/6
  NOT511/1 -> Logical Operator82/7
  NOT178/1 -> Logical Operator84/2
  NOT424/1 -> Logical Operator99/5
  NOT423/1 -> Logical Operator99/4
  NOT426/1 -> Logical Operator99/7
  NOT410/1 -> Logical Operator94/6
  NOT486/1 -> Logical Operator70/2
  NOT344/1 -> Logical Operator103/5
  NOT446/1 -> Logical Operator120/3
  NOT385/1 -> Logical Operator87/5
  NOT445/1 -> Logical Operator120/2
  NOT493/1 -> Logical Operator65/2
  NOT322/1 -> Logical Operator76/4
  NOT320/1 -> Logical Operator79/6
  NOT491/1 -> Logical Operator71/3
  NOT331/1 -> Logical Operator76/5
  NOT447/1 -> Logical Operator120/4
  NOT373/1 -> Logical Operator118/7
  NOT369/1 -> Logical Operator118/4
  NOT376/1 -> Logical Operator87/4
  NOT254/1 -> Logical Operator65/6
  NOT293/1 -> Logical Operator89/7
  NOT372/1 -> Logical Operator73/4
  NOT109/1 -> Logical Operator64/2
  NOT346/1 -> Logical Operator102/3
  NOT405/1 -> Logical Operator93/3
  NOT403/1 -> Logical Operator98/2
  NOT362/1 -> Logical Operator73/3
  NOT441/1 -> Logical Operator109/3
  NOT301/1 -> Logical Operator76/2
  NOT384/1 -> Logical Operator122/3
  NOT471/1 -> Logical Operator64/7
  NOT227/1 -> Logical Operator85/6
  NOT481/1 -> Logical Operator68/6
  NOT416/1 -> Logical Operator95/6
  NOT500/1 -> Logical Operator72/7
  NOT450/1 -> Logical Operator125/2
  NOT483/1 -> Logical Operator68/7
  NOT453/1 -> Logical Operator125/4
  NOT304/1 -> Logical Operator112/6
  NOT290/1 -> Logical Operator89/5
  NOT357/1 -> Logical Operator64/3
  NOT332/1 -> Logical Operator116/5
  NOT506/1 -> Logical Operator82/2
  NOT311/1 -> Logical Operator76/3
  NOT438/1 -> Logical Operator64/4
  NOT364/1 -> Logical Operator114/4
  NOT421/1 -> Logical Operator98/4
  NOT313/1 -> Logical Operator79/2
  NOT452/1 -> Logical Operator125/3
  NOT499/1 -> Logical Operator72/6
  In3/1 -> NOT9/1, NOT21/1, NOT26/1, NOT32/1, NOT42/1, NOT46/1, NOT57/1, NOT75/1, NOT78/1, Logical Operator16/3, Logical Operator18/3, Logical Operator27/3, Logical Operator28/3, Logical Operator30/3, Logical Operator31/3, Logical Operator32/3, Logical Operator19/3, Logical Operator21/3, Logical Operator23/3, Logical Operator24/3, NOT187/1, NOT211/1, NOT229/1, NOT233/1, NOT245/1, NOT251/1, NOT261/1, NOT268/1, Logical Operator40/3, Logical Operator49/3, Logical Operator51/3, Logical Operator53/3, Logical Operator56/3, Logical Operator42/3, Logical Operator44/3, Logical Operator45/3, Logical Operator46/3, Logical Operator47/3, NOT503/1, NOT311/1, NOT367/1, NOT441/1, NOT446/1, NOT456/1, NOT463/1, NOT478/1, NOT488/1, NOT491/1, Logical Operator74/3, Logical Operator82/3, Logical Operator84/3, Logical Operator85/3, Logical Operator86/3, Logical Operator89/3, Logical Operator77/3, Logical Operator79/3, NOT362/1, NOT429/1, NOT346/1, NOT368/1, NOT374/1, NOT388/1, NOT395/1, NOT399/1, NOT408/1, NOT419/1, Logical Operator100/3, Logical Operator108/3, Logical Operator110/3, Logical Operator111/3, Logical Operator112/3, Logical Operator115/3, Logical Operator101/3, Logical Operator103/3, Logical Operator104/3, Logical Operator105/3, Logical Operator106/3, Logical Operator107/3, Logical Operator117/3, Logical Operator116/3, Logical Operator113/3, Logical Operator99/3, NOT417/1, NOT414/1, NOT405/1, NOT384/1, NOT379/1, NOT363/1, Logical Operator81/3, Logical Operator80/3, Logical Operator78/3, Logical Operator75/3, Logical Operator90/3, Logical Operator88/3, Logical Operator83/3, Logical Operator72/3, NOT484/1, NOT474/1, NOT468/1, NOT452/1, NOT412/1, NOT357/1, Logical Operator48/3, Logical Operator57/3, Logical Operator55/3, Logical Operator52/3, Logical Operator50/3, Logical Operator41/3, NOT265/1, NOT255/1, NOT240/1, NOT223/1, NOT218/1, NOT206/1, NOT279/1, NOT204/1, Logical Operator22/3, Logical Operator20/3, Logical Operator29/3, Logical Operator26/3, Logical Operator25/3, NOT71/1, NOT66/1, NOT62/1, NOT52/1, NOT37/1, NOT15/1, NOT2/1
  In4/1 -> NOT10/1, NOT22/1, NOT27/1, NOT33/1, NOT38/1, NOT43/1, Logical Operator11/4, Logical Operator12/4, Logical Operator13/4, Logical Operator14/4, NOT88/1, NOT94/1, NOT113/1, NOT118/1, Logical Operator31/4, Logical Operator20/4, Logical Operator23/4, Logical Operator24/4, NOT93/1, NOT196/1, NOT224/1, NOT230/1, Logical Operator62/4, Logical Operator63/4, Logical Operator34/4, Logical Operator39/4, NOT273/1, NOT283/1, NOT98/1, NOT112/1, NOT134/1, NOT149/1, Logical Operator57/4, Logical Operator44/4, Logical Operator45/4, Logical Operator47/4, NOT438/1, NOT131/1, NOT322/1, NOT376/1, NOT421/1, NOT447/1, NOT453/1, Logical Operator127/4, Logical Operator67/4, Logical Operator68/4, Logical Operator71/4, NOT497/1, NOT244/1, NOT272/1, Logical Operator78/4, Logical Operator79/4, Logical Operator81/4, NOT372/1, NOT507/1, NOT354/1, NOT364/1, NOT375/1, Logical Operator123/4, Logical Operator124/4, Logical Operator96/4, Logical Operator97/4, NOT433/1, NOT512/1, NOT295/1, NOT310/1, NOT328/1, Logical Operator117/4, Logical Operator101/4, Logical Operator103/4, Logical Operator104/4, Logical Operator105/4, Logical Operator106/4, Logical Operator107/4, Logical Operator116/4, NOT210/1, NOT427/1, NOT423/1, Logical Operator95/4, Logical Operator94/4, Logical Operator93/4, Logical Operator92/4, NOT386/1, NOT380/1, NOT369/1, Logical Operator80/4, Logical Operator77/4, Logical Operator75/4, Logical Operator90/4, Logical Operator89/4, NOT217/1, NOT182/1, NOT162/1, NOT508/1, NOT501/1, Logical Operator70/4, Logical Operator69/4, Logical Operator66/4, Logical Operator126/4, NOT442/1, Logical Operator48/4, Logical Operator46/4, Logical Operator42/4, Logical Operator56/4, NOT166/1, NOT277/1, Logical Operator38/4, Logical Operator37/4, Logical Operator36/4, Logical Operator35/4, NOT219/1, NOT212/1, NOT207/1, NOT215/1, Logical Operator22/4, Logical Operator21/4, Logical Operator19/4, Logical Operator32/4, NOT124/1, NOT106/1, NOT101/1, NOT83/1, Logical Operator15/4, Logical Operator10/4, Logical Operator9/4, Logical Operator8/4, NOT16/1, NOT3/1
  In6/1 -> Logical Operator2/6, Logical Operator7/6, Logical Operator14/6, NOT85/1, Logical Operator25/6, NOT115/1, Logical Operator30/6, NOT130/1, NOT137/1, Logical Operator19/6, Logical Operator20/6, NOT237/1, NOT159/1, Logical Operator43/6, Logical Operator61/6, Logical Operator35/6, Logical Operator38/6, Logical Operator39/6, NOT275/1, NOT280/1, Logical Operator50/6, NOT177/1, Logical Operator47/6, NOT254/1, Logical Operator76/6, Logical Operator87/6, NOT437/1, Logical Operator66/6, Logical Operator67/6, Logical Operator70/6, Logical Operator82/6, NOT194/1, NOT227/1, NOT292/1, Logical Operator75/6, Logical Operator77/6, NOT314/1, Logical Operator80/6, NOT392/1, Logical Operator102/6, Logical Operator114/6, NOT378/1, Logical Operator122/6, NOT391/1, NOT410/1, NOT416/1, Logical Operator96/6, Logical Operator97/6, NOT425/1, NOT431/1, Logical Operator108/6, Logical Operator110/6, NOT257/1, Logical Operator113/6, Logical Operator115/6, Logical Operator101/6, NOT349/1, Logical Operator106/6, Logical Operator107/6, NOT353/1, Logical Operator103/6, NOT338/1, NOT334/1, NOT304/1, Logical Operator93/6, Logical Operator92/6, NOT398/1, Logical Operator121/6, NOT371/1, NOT321/1, Logical Operator81/6, NOT320/1, NOT298/1, Logical Operator88/6, Logical Operator86/6, Logical Operator83/6, NOT504/1, NOT499/1, Logical Operator71/6, NOT487/1, NOT481/1, NOT466/1, NOT459/1, Logical Operator125/6, Logical Operator120/6, NOT444/1, NOT460/1, Logical Operator48/6, NOT195/1, NOT190/1, Logical Operator44/6, Logical Operator42/6, NOT172/1, Logical Operator55/6, Logical Operator53/6, NOT142/1, NOT120/1, Logical Operator49/6, NOT264/1, NOT258/1, Logical Operator34/6, NOT243/1, NOT236/1, Logical Operator60/6, NOT221/1, NOT214/1, Logical Operator54/6, Logical Operator24/6, Logical Operator23/6, NOT158/1, NOT152/1, Logical Operator29/6, NOT108/1, Logical Operator26/6, NOT90/1, Logical Operator15/6, NOT74/1, NOT69/1, Logical Operator11/6, Logical Operator10/6, NOT55/1, NOT49/1, Logical Operator6/6, NOT35/1, NOT29/1, Logical Operator3/6, NOT12/1, NOT5/1
  Logical Operator/1 -> 0000000/1
  Logical Operator1/1 -> "0000001 "/1
  Logical Operator2/1 -> 0000010/1
  Logical Operator3/1 -> 0000011/1
  Logical Operator4/1 -> 0000100/1
  Logical Operator5/1 -> 0000101/1
  Logical Operator6/1 -> 0000110/1
  Logical Operator7/1 -> 0000111/1
  Logical Operator8/1 -> 0001000/1
  Logical Operator9/1 -> 0001001/1
  Logical Operator10/1 -> 0001010/1
  Logical Operator11/1 -> 0001011/1
  Logical Operator12/1 -> 0001100/1
  Logical Operator13/1 -> 0001101/1
  Logical Operator14/1 -> 0001110/1
  Logical Operator15/1 -> 0001111/1
  Logical Operator16/1 -> 0010000/1
  Logical Operator18/1 -> 0010001/1
  Logical Operator26/1 -> 0010011/1
  Logical Operator25/1 -> 0010010/1
  Logical Operator27/1 -> 0010100/1
  Logical Operator28/1 -> 0010101/1
  Logical Operator29/1 -> 0010110/1
  Logical Operator30/1 -> 0010111/1
  Logical Operator31/1 -> 0011000/1
  Logical Operator19/1 -> 0011010/1
  Logical Operator32/1 -> 0011001/1
  Logical Operator20/1 -> 0011011/1
  Logical Operator21/1 -> 0011100/1
  Logical Operator22/1 -> 0011101/1
  Logical Operator23/1 -> 0011110/1
  Logical Operator24/1 -> 0011111/1
  Logical Operator17/1 -> 0100000/1
  Logical Operator33/1 -> 0100001/1
  Logical Operator43/1 -> 0100010/1
  Logical Operator58/1 -> 0100100/1
  Logical Operator54/1 -> 0100011/1
  Logical Operator59/1 -> 0100101/1
  Logical Operator60/1 -> 0100110/1
  Logical Operator61/1 -> 0100111/1
  Logical Operator63/1 -> 0101001/1
  Logical Operator62/1 -> 0101000/1
  Logical Operator34/1 -> 0101010/1
  Logical Operator35/1 -> 0101011/1
  Logical Operator36/1 -> 0101100/1
  Logical Operator37/1 -> 0101101/1
  Logical Operator38/1 -> 0101110/1
  Logical Operator39/1 -> 0101111/1
  Logical Operator40/1 -> 0110000/1
  Logical Operator41/1 -> 0110001/1
  Logical Operator49/1 -> 0110010/1
  Logical Operator50/1 -> 0110011/1
  Logical Operator51/1 -> 0110100/1
  Logical Operator52/1 -> 0110101/1
  Logical Operator53/1 -> 0110110/1
  Logical Operator55/1 -> 0110111/1
  Logical Operator56/1 -> 0111000/1
  Logical Operator57/1 -> 0111001/1
  Logical Operator42/1 -> 0111010/1
  Logical Operator44/1 -> 0111011/1
  Logical Operator45/1 -> 0111100/1
  Logical Operator46/1 -> 0111101/1
  Logical Operator47/1 -> 0111110/1
  Logical Operator48/1 -> 0111111/1
  Logical Operator64/1 -> 1000000/1
  Logical Operator65/1 -> 1000001/1
  Logical Operator76/1 -> 1000010/1
  Logical Operator87/1 -> 1000011/1
  Logical Operator98/1 -> 1000100/1
  Logical Operator120/1 -> 1000110/1
  Logical Operator109/1 -> 1000101/1
  Logical Operator125/1 -> 1000111/1
  Logical Operator126/1 -> 1001000/1
  Logical Operator127/1 -> 1001001/1
  Logical Operator66/1 -> 1001010/1
  Logical Operator67/1 -> 1001011/1
  Logical Operator68/1 -> 1001100/1
  Logical Operator69/1 -> 1001101/1
  Logical Operator70/1 -> 1001110/1
  Logical Operator71/1 -> 1001111/1
  Logical Operator72/1 -> 1010000/1
  Logical Operator74/1 -> 1010001/1
  Logical Operator82/1 -> 1010010/1
  Logical Operator83/1 -> 1010011/1
  Logical Operator84/1 -> 1010100/1
  Logical Operator85/1 -> 1010101/1
  Logical Operator86/1 -> 1010110/1
  Logical Operator88/1 -> 1010111/1
  Logical Operator89/1 -> 1011000/1
  Logical Operator90/1 -> 1011001/1
  Logical Operator75/1 -> 1011010/1
  Logical Operator77/1 -> 1011011/1
  Logical Operator78/1 -> "1011100 "/1
  Logical Operator79/1 -> 1011101/1
  Logical Operator80/1 -> 1011110/1
  Logical Operator81/1 -> 1011111/1
  Logical Operator73/1 -> 1100000/1
  Logical Operator91/1 -> 1100001/1
  Logical Operator102/1 -> 1100010/1
  Logical Operator114/1 -> 1100011/1
  Logical Operator118/1 -> 1100100/1
  Logical Operator119/1 -> 1100101/1
  Logical Operator121/1 -> 1100110/1
  Logical Operator122/1 -> 1100111/1
  Logical Operator123/1 -> 1101000/1
  Logical Operator124/1 -> 1101001/1
  Logical Operator92/1 -> 1101010/1
  Logical Operator93/1 -> 1101011/1
  Logical Operator94/1 -> 1101100/1
  Logical Operator95/1 -> 1101101/1
  Logical Operator96/1 -> 1101110/1
  Logical Operator97/1 -> 1101111/1
  Logical Operator99/1 -> 1110000/1
  Logical Operator100/1 -> 1110001/1
  Logical Operator108/1 -> 1110010/1
  Logical Operator110/1 -> 1110011/1
  Logical Operator111/1 -> 1110100/1
  Logical Operator112/1 -> 1110101/1
  Logical Operator113/1 -> 1110110/1
  Logical Operator115/1 -> 1110111/1
  Logical Operator116/1 -> 1111000/1
  Logical Operator117/1 -> 1111001/1
  Logical Operator101/1 -> 1111010/1
  Logical Operator103/1 -> 1111011/1
  Logical Operator104/1 -> 1111100/1
  Logical Operator105/1 -> 1111101/1
  Logical Operator106/1 -> 1111110/1
  Logical Operator107/1 -> 1111111/1

== system PONG/Horizontal Bounce ==
  Check : Inport
  CLK : Inport  Port=2
  J-K Flip-Flop : simulink_extras/Flip Flops/J-K Flip-Flop  initial_condition=0
      settings: SourceProductName=Simulink
  HEnable : Outport
  wires:
  Check/1 -> J-K Flip-Flop/1, J-K Flip-Flop/3
  J-K Flip-Flop/1 -> HEnable/1
  CLK/1 -> J-K Flip-Flop/2
